simulink model "AOR_Instant"  (R2016b)
settings: Solver=ode23tb  StartTime=0.0  StopTime=35  MaxStep=0.01  RelTol=1e-3
values from neighbouring files (symbols this model uses):
  A = [3 1;-1 0]    [Init_AOR.m]
  Al = [1;0]    [Init_AOR.m]
  As = [20,60]    [Init_AOR.m]
  B = [1;1]    [Init_AOR.m]
  C = [1 0]    [Init_AOR.m]
  D = 0    [Init_AOR.m]
  E = zeros(2,4)    [Init_AOR.m]
  F = -R    [Init_AOR.m]
  G = [750 2500 5 100]    [Init_AOR.m]
  L = [1 2*p p]    [Init_AOR.m]
  mu = 100    [Init_AOR.m]
  P = [-2, -6]    [Init_AOR.m]
  R = [1 0 0 0]    [Init_AOR.m]
  S = [0 w1 0 0;-w1 0 0 0;0 0 0 w2;0 0 -w2 0]    [Init_AOR.m]
  t0 = ones(4,1)    [Init_AOR.m]
  V0 = [1 0 1 0]'    [Init_AOR.m]
  X0 = ones(2,1)    [Init_AOR.m]
  Z0 = ones(3*n,1)    [Init_AOR.m]
settings Model: Creator=Niels  LastModifiedBy=Niels
settings SolverCC: ZeroCrossAlgorithm=Adaptive

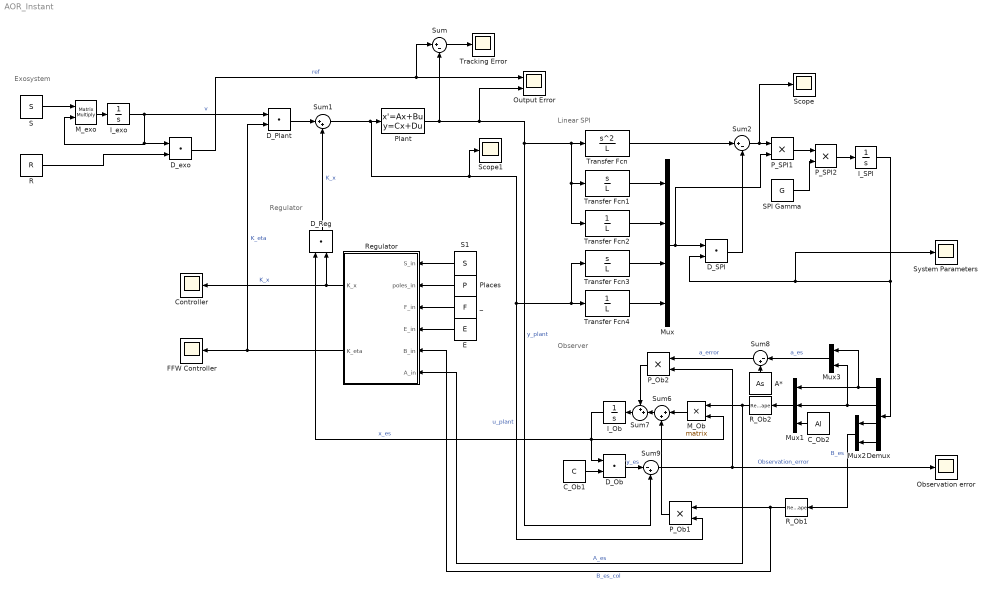
== system AOR_Instant ==
  note: Exosystem
  note: Regulator
  note: Observer
  note: Linear SPI
  "A* " : Constant  Value=As
  C_Ob1 : Constant  Value=C
  C_Ob2 : Constant  Value=Al
  Controller : Scope
  D_Ob : DotProduct  InputSameDT=on  OutDataTypeStr=Inherit: Inherit via internal rule
  D_Plant : DotProduct  InputSameDT=on  OutDataTypeStr=Inherit: Inherit via internal rule
  "D_Reg " : DotProduct  InputSameDT=on  OutDataTypeStr=Inherit: Inherit via internal rule
  D_SPI : DotProduct  InputSameDT=on  OutDataTypeStr=Inherit: Inherit via internal rule
  D_exo : DotProduct  InputSameDT=on  OutDataTypeStr=Inherit: Inherit via internal rule
  Demux : Demux
  E : Constant  Value=E
  FFW Controller : Scope
  I_Ob : Integrator  InitialCondition=X0
  I_SPI : Integrator  InitialCondition=t0
  I_exo : Integrator  InitialCondition=V0
  M_Ob : Product  Multiplication=Matrix(*)
  M_exo : Product  Inputs=**  Multiplication=Matrix(*)
  Mux : Mux
  Mux1 : Mux  Inputs=3
  Mux2 : Mux  Inputs=2
  Mux3 : Mux  Inputs=2
  Observation error : Scope
  Output Error : Scope  NumInputPorts=2
  P_Ob1 : Product
  P_Ob2 : Product
  P_SPI1 : Product
  P_SPI2 : Product
  Places : Constant  Value=P  VectorParams1D=off
  Plant : StateSpace  A=A  B=B  C=C  D=D  X0=0
  R : Constant  Value=R  VectorParams1D=off
  R_Ob1 : Reshape  OutputDimensionality=Customize  OutputDimensions=[2,1]
  R_Ob2 : Reshape  OutputDimensionality=Customize  OutputDimensions=[2,2]
  Regulator : Subsystem
  S : Constant  Value=S
  S1 : Constant  Value=S
  SPI Gamma : Constant  Value=G
  Scope : Scope
  Scope1 : Scope
  Sum : Sum  Inputs=|+-
  Sum1 : Sum  Inputs=|++
  Sum2 : Sum  Inputs=|+-
  Sum6 : Sum  Inputs=|++
  Sum7 : Sum  Inputs=++|
  Sum8 : Sum  Inputs=|-+
  Sum9 : Sum  Inputs=|-+
  "System Parameters " : Scope
  Tracking Error : Scope
  Transfer Fcn : TransferFcn  Numerator=[1 0 0]  Denominator=L
  Transfer Fcn1 : TransferFcn  Numerator=[1 0 ]  Denominator=L
  Transfer Fcn2 : TransferFcn  Denominator=L
  Transfer Fcn3 : TransferFcn  Numerator=[1 0 ]  Denominator=L
  Transfer Fcn4 : TransferFcn  Denominator=L
  _ : Constant  Value=F  VectorParams1D=off
  wires:
  Transfer Fcn1/1 -> Mux/1
  Transfer Fcn2/1 -> Mux/2
  Transfer Fcn3/1 -> Mux/3
  Transfer Fcn4/1 -> Mux/4
  Mux/1 -> D_SPI/1, P_SPI1/2
  Transfer Fcn/1 -> Sum2/1
  D_SPI/1 -> Sum2/2
  Sum2/1 -> Scope/1, P_SPI1/1
  P_SPI1/1 -> P_SPI2/1
  SPI Gamma/1 -> P_SPI2/2
  P_SPI2/1 -> I_SPI/1
  Sum1/1 -> Scope1/1, Transfer Fcn4/1, Transfer Fcn3/1, P_Ob1/2, Plant/1  "u_plant"
  Demux/1 -> Mux3/1, Mux1/1
  Demux/2 -> Mux3/2, Mux1/2
  Mux1/1 -> R_Ob2/1
  C_Ob2/1 -> Mux1/3
  R_Ob2/1 -> M_Ob/1, Regulator/6(A_in)  "A_es"
  Demux/4 -> Mux2/2
  Demux/3 -> Mux2/1
  Mux2/1 -> R_Ob1/1  "B_es"
  Plant/1 -> Sum/2, Sum9/2, Transfer Fcn2/1, Transfer Fcn1/1, Transfer Fcn/1, Output Error/2  "y_plant"
  M_Ob/1 -> Sum6/1
  Sum6/1 -> Sum7/2
  Sum7/1 -> I_Ob/1
  I_Ob/1 -> "D_Reg "/1, M_Ob/2, D_Ob/1  "x_es"
  P_Ob1/1 -> Sum6/2
  Sum8/1 -> P_Ob2/1  "a_error"
  C_Ob1/1 -> D_Ob/2
  Sum9/1 -> Observation error/1, P_Ob2/2  "Observation_error"
  D_Ob/1 -> Sum9/1  "y_es"
  Mux3/1 -> Sum8/1  "a_es"
  "A* "/1 -> Sum8/2
  P_Ob2/1 -> Sum7/1
  D_Plant/1 -> Sum1/1
  Regulator/1(K_x) -> Controller/1, "D_Reg "/2  "K_x"
  "D_Reg "/1 -> Sum1/2  "K_x"
  Regulator/2(K_eta) -> D_Plant/2, FFW Controller/1  "K_eta"
  M_exo/1 -> I_exo/1
  I_exo/1 -> D_Plant/1, M_exo/2, D_exo/1  "v"
  S/1 -> M_exo/1
  R/1 -> D_exo/2
  E/1 -> Regulator/4(E_in)
  S1/1 -> Regulator/1(S_in)
  Places/1 -> Regulator/2(poles_in)
  _/1 -> Regulator/3(F_in)
  R_Ob1/1 -> Regulator/5(B_in), P_Ob1/1  "B_es_col"
  D_exo/1 -> Sum/1, Output Error/1  "ref"
  I_SPI/1 -> Demux/1, D_SPI/2, "System Parameters "/1
  Sum/1 -> Tracking Error/1

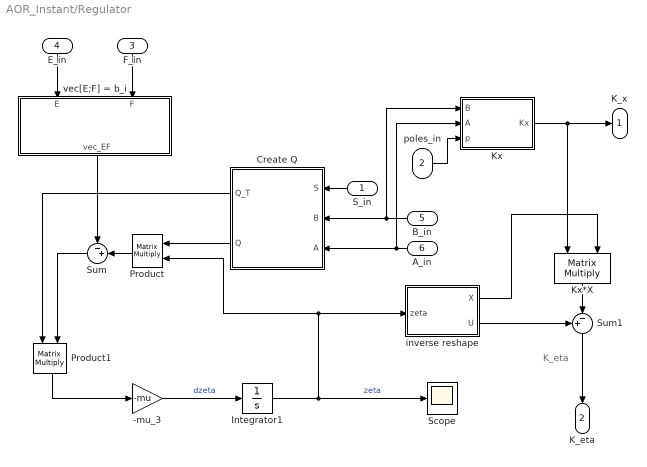
== system AOR_Instant/Regulator ==
  note: K_eta
  S_in : Inport
  poles_in : Inport  Port=2
  F_in : Inport  Port=3
  E_in : Inport  Port=4
  B_in : Inport  Port=5
  A_in : Inport  Port=6
  -mu_3 : Gain  Gain=-mu
  Create Q : MATLAB Function  TreatAsAtomicUnit=on
  Integrator1 : Integrator  InitialCondition=Z0
  Kx : MATLAB Function  TreatAsAtomicUnit=on
  Kx*X : Product  Inputs=**  Multiplication=Matrix(*)
  Product : Product  Multiplication=Matrix(*)
  Product1 : Product  Multiplication=Matrix(*)
  Scope : Scope
  Sum : Sum  Inputs=-+|
  Sum1 : Sum  Inputs=+-|
  inverse reshape : MATLAB Function  TreatAsAtomicUnit=on
  "vec[E;F] = b_i   " : MATLAB Function  TreatAsAtomicUnit=on
  K_x : Outport
  K_eta : Outport  Port=2
  wires:
  inverse reshape/1(X) -> Kx*X/2
  inverse reshape/2(U) -> Sum1/1
  F_in/1 -> "vec[E;F] = b_i   "/2(F)
  Create Q/2(Q) -> Product/1
  Product1/1 -> -mu_3/1
  Sum1/1 -> K_eta/1
  Sum/1 -> Product1/2
  Create Q/1(Q_T) -> Product1/1
  Kx*X/1 -> Sum1/2
  poles_in/1 -> Kx/3(p)
  Integrator1/1 -> Scope/1, inverse reshape/1(zeta), Product/2  "zeta"
  -mu_3/1 -> Integrator1/1  "dzeta"
  Kx/1(Kx) -> Kx*X/1, K_x/1
  S_in/1 -> Create Q/1(S)
  A_in/1 -> Create Q/3(A), Kx/2(A)
  B_in/1 -> Kx/1(B), Create Q/2(B)
  E_in/1 -> "vec[E;F] = b_i   "/1(E)
  "vec[E;F] = b_i   "/1(vec_EF) -> Sum/1
  Product/1 -> Sum/2

== matlab function AOR_Instant/Regulator/Create Q ==
  data: Q_T output size=[3*n,3*n]; Q output size=[3*n,3*n]; S input; B input; A input
function [Q_T,Q]= fcn(S,B,A)
[Sc,Sr]=size(S);
I_ni = [eye(2) zeros(2,1);zeros(1,3)];
I_q = eye(Sc);
sysmatrix = [A B;1 0 0];

Q = kron(S.',I_ni)-kron(I_q,sysmatrix);
Q_T = Q.';
end

== matlab function AOR_Instant/Regulator/Kx ==
  data: B input; A input; Kx output; p input
function Kx = fcn(B,A,p)

coder.extrinsic('place')
Kx = zeros(1,2);
Kx = place(A,-B,p);

== matlab function AOR_Instant/Regulator/inverse reshape ==
  data: zeta input; X output; U output
function [X,U] = fcn(zeta)
n = 4;
tmp = reshape(zeta,3,n);
X = tmp(1:2,1:n);
U = tmp(3,:);
end

== matlab function AOR_Instant/Regulator/vec[E;F] = b_i    ==
  data: E input; vec_EF output; F input
function vec_EF = fcn(E,F)
[Ec,Er] = size(E);
[Fc,Fr] = size(F);
vec_EF = reshape([E;F],Ec*Er+Fc*Fr,1);
end
